simulink model "CurBasedFluxEst_sim"  (R2021b)
settings: Solver=FixedStepAuto  StartTime=0.0  StopTime=SimTime  FixedStep=Ts_sim  MaxStep=Ts_sim  RelTol=1e-3
values from neighbouring files (symbols this model uses):
  FstoWm = 1/PolePairs * 2 * pi    (= 3.14159265359)    [CurBasedFluxEst_param.m]
  Llr = 0.005473    [CurBasedFluxEst_param.m]
  NsToFs = PolePairs/60    (= 0.0333333333333)    [CurBasedFluxEst_param.m]
  PolePairs = 2    [CurBasedFluxEst_param.m]
  RotFluxEst_Ts = Ts_sim    (= 1e-06)    [CurBasedFluxEst_param.m]
  Rr = 0.6258    [CurBasedFluxEst_param.m]
  SVPWM_SampTs = 1/SVPWM_SampFreq    (= 0.001)    [CurBasedFluxEst_param.m]
  SVPWM_SwitchTs = 1/SVPWM_SwitchFreq    (= 5e-05)    [CurBasedFluxEst_param.m]
  Test_NsCntr = 6    [CurBasedFluxEst_param.m]
  Test_NsMax = max(Test_NsArr)    [CurBasedFluxEst_param.m]
  Test_wTs = 1    [CurBasedFluxEst_param.m]
  Tr = Lr / Rr    (= 0.0653131991051)    [CurBasedFluxEst_param.m]
  Ts_sim = 1e-6    (= 1e-06)    [CurBasedFluxEst_param.m]
  Udc = 400    [CurBasedFluxEst_param.m]
  UFCtrl_FWPointFreq = NomFreq    (= 60)    [CurBasedFluxEst_param.m]
  UFCtrl_LinRegPointFreq = 5    [CurBasedFluxEst_param.m]
  UFCtrl_MaxFreq = UFCtrl_FWPointFreq * 2    (= 120)    [CurBasedFluxEst_param.m]
  UFCtrl_Ts = Ts_sim    (= 1e-06)    [CurBasedFluxEst_param.m]
  UFCtrl_UBelowLinReg = 5    [CurBasedFluxEst_param.m]
  UNomLL = 400    [CurBasedFluxEst_param.m]
undefined symbols (not defined in the file or in its folder): NsCntr, Ts_stair
libraries: spsIGBTDiodeLib x6, spsCurrentMeasurementLib x3, spsVoltageMeasurementLib x3, simulink x2, spsAsynchronousMachineSIUnitsLib x1, spsDCVoltageSourceLib x1, spspowerguiLib x1
settings Model: Creator=ArnóczyLászlóVince  LastModifiedBy=ArnóczyLászlóVince

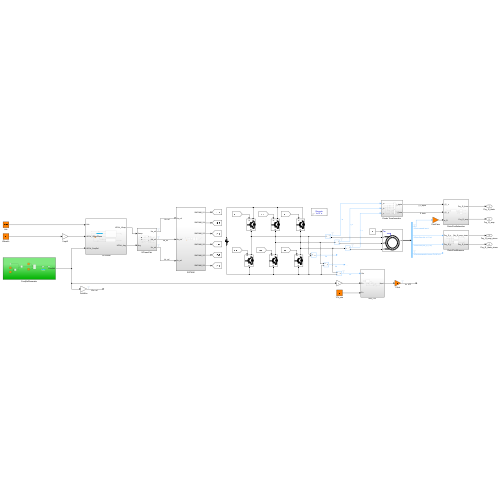
[thumbnail: Simulink's stored preview of the top-level diagram]
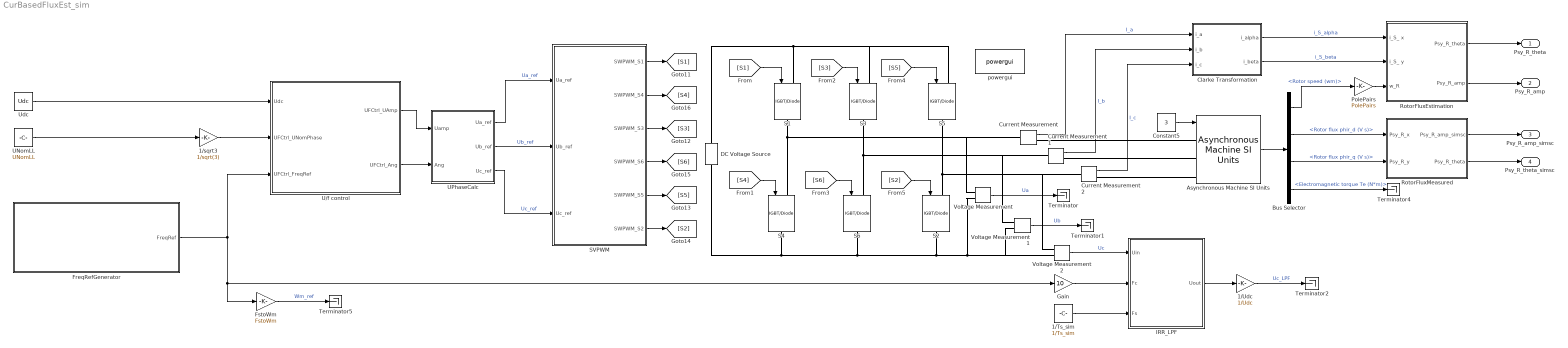
== system CurBasedFluxEst_sim ==
  1/Ts_sim : Constant  Value=1/Ts_sim
  1/Udc : Gain  Gain=1/Udc
  1/sqrt3 : Gain  Gain=1/sqrt(3)
  Asynchronous Machine SI Units : spsAsynchronousMachineSIUnitsLib/Asynchronous Machine SI Units  RotorType=Squirrel-cage  PresetModel=No  MechanicalLoad=Torque Tm  ShowDetailedParameters=on  ReferenceFrame=Stationary  Units=SI  MeasurementBus=off  NominalParameters=[1.845e+04 400 60]  VoltageRatio=1  Stator=[0.5968 0.0003495]  Rotor=[Rr Llr]  Cage1=[0.4155 0.002066]  Cage2=[0.4168 0.0003495]  Lm=Lm  Mechanical=[0.05 0.005879 PolePairs]  PolePairs=PolePairs  InitialConditions=[0 0 0 0 0 0 0 0]  SimulateSaturation=off  Saturation=[14.03593122, 27.81365428, 53.79336849, 72.68890987, 97.98006896, 148.6815601, 215.7428561, 302.9841135, 428.7778367 ; 230, 322, 414, 460, 506, 552, 598, 644, 690]  LoadFlowParameters=1492000  TsPowergui=0  TsBlock=-1  IterativeModel=Trapezoidal non iterative  IterativeDiscreteModel=Trapezoidal non iterative  Pmec=1.492e+006
  Bus Selector : BusSelector  OutputSignals=Mechanical.Rotor speed (wm),Rotor measurements.Rotor flux phir_d (V s),Rotor measurements.Rotor flux phir_q (V s),Mechanical.Electromagnetic torque Te (N*m)
  Clarke Transformation : Subsystem
  Constant5 : Constant  Value=3
  Current Measurement : spsCurrentMeasurementLib/Current Measurement  PhasorSimulation=off  OutputType=Complex  PSBequivalent=0
  Current Measurement1 : spsCurrentMeasurementLib/Current Measurement  PhasorSimulation=off  OutputType=Complex  PSBequivalent=0
  Current Measurement2 : spsCurrentMeasurementLib/Current Measurement  PhasorSimulation=off  OutputType=Complex  PSBequivalent=0
  DC Voltage Source : spsDCVoltageSourceLib/DC Voltage Source  Amplitude=Udc  Measurements=None
  FreqRefGenerator : Subsystem
  FstoWm : Gain  Gain=FstoWm
  Gain : Gain  Gain=10
  IRR_LPF : Subsystem
  PolePairs : Gain  Gain=PolePairs
  RotorFluxEstimation : Subsystem
  RotorFluxMeasured : Subsystem
  S{1..6} (6 alike) : spsIGBTDiodeLib/IGBT//Diode  Ron=1e-3  Rs=1e5  Cs=inf  Measurements=off
  SVPWM : Subsystem
  Terminator{,1..2,4..5} (5 alike) : Terminator
  U/f control : Subsystem
  UNomLL : Constant  Value=UNomLL
  UPhaseCalc : Subsystem
  Udc : Constant  Value=Udc
  Voltage Measurement : spsVoltageMeasurementLib/Voltage Measurement  PhasorSimulation=off  OutputType=Complex  PSBequivalent=0
  Voltage Measurement1 : spsVoltageMeasurementLib/Voltage Measurement  PhasorSimulation=off  OutputType=Complex  PSBequivalent=0
  Voltage Measurement2 : spsVoltageMeasurementLib/Voltage Measurement  PhasorSimulation=off  OutputType=Complex  PSBequivalent=0
  powergui : spspowerguiLib/powergui  Priority=1  SimulationMode=Discrete  SampleTime=Ts_sim  frequency=60  Iterations=50  frequencyindice=0  Pbase=100e6  ErrMax=1e-4  UnitsV=kV  UnitsW=MW  buscounter=0  FunctionMessages=off  echomessages=off  EnableUseOfTLC=off  CurrentSourceSwitches=off  DisableSnubberDevices=off  DisableRonSwitches=off  DisableVfSwitches=off  DisplayEquations=off  AutomaticDiscreteSolvers=off  SolverType=Tustin/Backward Euler (TBE)  Interpol=off  ExternalGateDelay=off  methode=off  Ts=100  x0status=blocks  SPID=on  SwTol=0  HookPort=off  NonlinearTolerance=1e-4  nMaxIteration=100  ContinueOnMaxIteration=off  RestoreLinks=warning  ResistiveCurrentMeasurement=off  Frange=[0:2:500]  Ylog=off  Xlog=on  ShowGrid=off  save=off  variable=ZData  structure=0  ZoomFFT=off  StartTime=0.0  cycles=1  DisplayStyle=1  fundamental=60  FreqAxis=off  MaxFrequency=1000  frequencyindicesteady=1  RmsSteady=1  display=off
  Psy_R_theta : Outport
  Psy_R_amp : Outport  Port=2
  Psy_R_amp_simsc : Outport  Port=3
  Psy_R_theta_simsc : Outport  Port=4
  wires:
  Clarke Transformation/1(i_alpha) -> RotorFluxEstimation/1(i_S_ x)  "i_S_alpha"
  Clarke Transformation/2(i_beta) -> RotorFluxEstimation/2(i_S_ y)  "i_S_beta"
  RotorFluxEstimation/1(Psy_R_theta) -> Psy_R_theta/1
  RotorFluxEstimation/2(Psy_R_amp) -> Psy_R_amp/1
  Asynchronous Machine SI Units/1 -> Bus Selector/1
  Current Measurement/1 -> Clarke Transformation/1(i_a)  "I_a"
  Current Measurement1/1 -> Clarke Transformation/2(i_b)  "I_b"
  Current Measurement2/1 -> Clarke Transformation/3(i_c)  "I_c"
  Bus Selector/1 -> PolePairs/1  "<Rotor speed (wm)>"
  [S1] -> S1/1
  [S4] -> S4/1
  [S3] -> S3/1
  [S6] -> S6/1
  [S5] -> S5/1
  [S2] -> S2/1
  Constant5/1 -> Asynchronous Machine SI Units/1
  Voltage Measurement2/1 -> IRR_LPF/1(Uin)  "Uc"
  Voltage Measurement1/1 -> Terminator1/1  "Ub"
  Voltage Measurement/1 -> Terminator/1  "Ua"
  SVPWM/1(SWPWM_S1) -> [S1]
  SVPWM/2(SWPWM_S4) -> [S4]
  SVPWM/3(SWPWM_S3) -> [S3]
  SVPWM/4(SWPWM_S6) -> [S6]
  SVPWM/5(SWPWM_S5) -> [S5]
  SVPWM/6(SWPWM_S2) -> [S2]
  PolePairs/1 -> RotorFluxEstimation/3(w_R)
  RotorFluxMeasured/1(Psy_R_amp_simsc) -> Psy_R_amp_simsc/1
  RotorFluxMeasured/2(Psy_R_theta) -> Psy_R_theta_simsc/1
  Bus Selector/3 -> RotorFluxMeasured/2(Psy_R_y)  "<Rotor flux phir_q (V s)>"
  Bus Selector/2 -> RotorFluxMeasured/1(Psy_R_x)  "<Rotor flux phir_d (V s)>"
  Bus Selector/4 -> Terminator4/1  "<Electromagnetic torque Te (N*m)>"
  UPhaseCalc/1(Ua_ref) -> SVPWM/1(Ua_ref)  "Ua_ref"
  UPhaseCalc/2(Ub_ref) -> SVPWM/2(Ub_ref)  "Ub_ref"
  UPhaseCalc/3(Uc_ref) -> SVPWM/3(Uc_ref)  "Uc_ref"
  UNomLL/1 -> 1/sqrt3/1
  FstoWm/1 -> Terminator5/1  "Wm_ref"
  U/f control/1(UFCtrl_UAmp) -> UPhaseCalc/1(Uamp)
  U/f control/2(UFCtrl_Ang) -> UPhaseCalc/2(Ang)
  1/sqrt3/1 -> U/f control/2(UFCtrl_UNomPhase)
  Udc/1 -> U/f control/1(Udc)
  FreqRefGenerator/1(FreqRef) -> U/f control/3(UFCtrl_FreqRef), FstoWm/1, Gain/1
  Gain/1 -> IRR_LPF/2(Fc)
  IRR_LPF/1(Uout) -> 1/Udc/1
  1/Udc/1 -> Terminator2/1  "Uc_LPF"
  1/Ts_sim/1 -> IRR_LPF/3(Fs)
  connections:
  Asynchronous Machine SI Units/LConn1 -- Current Measurement/RConn1
  S3/RConn1 -- Current Measurement1/LConn1 -- Voltage Measurement1/LConn1 -- S6/LConn1
  S4/LConn1 -- Current Measurement/LConn1 -- Voltage Measurement/LConn1 -- S1/RConn1
  S2/LConn1 -- Current Measurement2/LConn1 -- Voltage Measurement2/LConn1 -- S5/RConn1
  DC Voltage Source/RConn1 -- S1/LConn1 -- S3/LConn1 -- S5/LConn1
  DC Voltage Source/LConn1 -- Voltage Measurement2/LConn2 -- Voltage Measurement1/LConn2 -- Voltage Measurement/LConn2 -- S2/RConn1 -- S6/RConn1 -- S4/RConn1
  Asynchronous Machine SI Units/LConn3 -- Current Measurement2/RConn1
  Asynchronous Machine SI Units/LConn2 -- Current Measurement1/RConn1

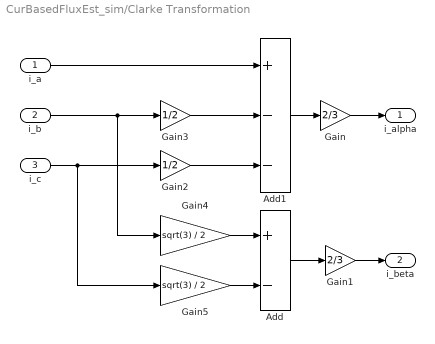
== system CurBasedFluxEst_sim/Clarke Transformation ==
  i_a : Inport
  i_b : Inport  Port=2
  i_c : Inport  Port=3
  Add : Sum  Inputs=+-
  Add1 : Sum  Inputs=+--
  Gain : Gain  Gain=2/3
  Gain1 : Gain  Gain=2/3
  Gain2 : Gain  Gain=1/2
  Gain3 : Gain  Gain=1/2
  Gain4 : Gain  Gain=sqrt(3) / 2
  Gain5 : Gain  Gain=sqrt(3) / 2
  i_alpha : Outport
  i_beta : Outport  Port=2
  wires:
  Gain4/1 -> Add/1
  Add/1 -> Gain1/1
  i_a/1 -> Add1/1
  Gain5/1 -> Add/2
  Add1/1 -> Gain/1
  Gain2/1 -> Add1/3
  Gain3/1 -> Add1/2
  i_b/1 -> Gain4/1, Gain3/1
  i_c/1 -> Gain5/1, Gain2/1
  Gain1/1 -> i_beta/1
  Gain/1 -> i_alpha/1

== system CurBasedFluxEst_sim/FreqRefGenerator ==
  note: Nr = ~ Ns
  Clock : Clock
  NrToFs : Gain  Gain=NsToFs
  Product : Product
  Relational Operator : RelationalOperator  OutDataTypeStr=boolean  RndMeth=Simplest
  Switch : Switch  Criteria=u2 ~= 0  Threshold=Ts_stair * NsCntr
  Test_NsArr : simulink/Sources/Repeating Sequence Stair  OutValues=Test_NsArr  tsamp=Test_wTs  OutMin=[]  OutMax=[]  OutDataTypeStr=double  OutputDataTypeScalingMode=double  OutDataType=fixdt(0,8)  ConRadixGroup=Best Precision: Vector-wise  OutScaling=2^-12
  Test_NsCntr : Constant  Value=Test_NsCntr
  Test_NsMax : Constant  Value=Test_NsMax
  Test_wTs : Constant  Value=Test_wTs
  FreqRef : Outport
  wires:
  Clock/1 -> Relational Operator/1
  Test_NsArr/1 -> Switch/3
  Test_NsCntr/1 -> Product/2
  Switch/1 -> NrToFs/1  "Nr_ref"
  Product/1 -> Relational Operator/2
  Test_NsMax/1 -> Switch/1
  Test_wTs/1 -> Product/1
  Relational Operator/1 -> Switch/2
  NrToFs/1 -> FreqRef/1

== system CurBasedFluxEst_sim/IRR_LPF ==
  Uin : Inport
  Fc : Inport  Port=2
  Fs : Inport  Port=3
  Add6 : Sum  Inputs=+-
  Add7 : Sum
  MATLAB Function : MATLAB Function  TreatAsAtomicUnit=on
  Product3 : Product
  Unit Delay3 : UnitDelay  SampleTime=-1  HasFrameUpgradeWarning=on
  Uout : Outport
  wires:
  Add6/1 -> Product3/2
  Product3/1 -> Add7/1
  MATLAB Function/1(alpha) -> Product3/1
  Unit Delay3/1 -> Add7/2, Add6/2
  Add7/1 -> Uout/1, Unit Delay3/1
  Uin/1 -> Add6/1
  Fc/1 -> MATLAB Function/1(Fc)
  Fs/1 -> MATLAB Function/2(Fs)

== system CurBasedFluxEst_sim/RotorFluxEstimation ==
  i_S_ x : Inport
  i_S_ y : Inport  Port=2
  w_R : Inport  Port=3
  PsyR_Amp_Calc : Subsystem
  PsyR_Amp_angle : Subsystem
  PsyR_XY_calc : Subsystem
  Psy_R_theta : Outport
  Psy_R_amp : Outport  Port=2
  wires:
  w_R/1 -> PsyR_XY_calc/2(w_R)
  i_S_ y/1 -> PsyR_XY_calc/3(i_S_ y)
  i_S_ x/1 -> PsyR_XY_calc/1(i_S_ x)
  PsyR_Amp_Calc/1(Psy_R_amp) -> Psy_R_amp/1
  PsyR_Amp_angle/1(Psy_R_theta) -> Psy_R_theta/1
  PsyR_XY_calc/1(Psy_R_ x) -> PsyR_Amp_Calc/1(Psy_R_ x), PsyR_Amp_angle/1(Psy_R_ x)
  PsyR_XY_calc/2(Psy_R_ y) -> PsyR_Amp_Calc/2(Psy_R_ y), PsyR_Amp_angle/2(Psy_R_ y)

== system CurBasedFluxEst_sim/RotorFluxMeasured ==
  Psy_R_x : Inport
  Psy_R_y : Inport  Port=2
  PsyR_Amp_Calc : Subsystem
  PsyR_Amp_angle : Subsystem
  Psy_R_amp_simsc : Outport
  Psy_R_theta : Outport  Port=2
  wires:
  PsyR_Amp_angle/1(Psy_R_theta) -> Psy_R_theta/1
  PsyR_Amp_Calc/1(Psy_R_amp_simsc) -> Psy_R_amp_simsc/1
  Psy_R_x/1 -> PsyR_Amp_Calc/1(Psy_x), PsyR_Amp_angle/1(Psy_R_ x)
  Psy_R_y/1 -> PsyR_Amp_Calc/2(Psy_y), PsyR_Amp_angle/2(Psy_R_ y)

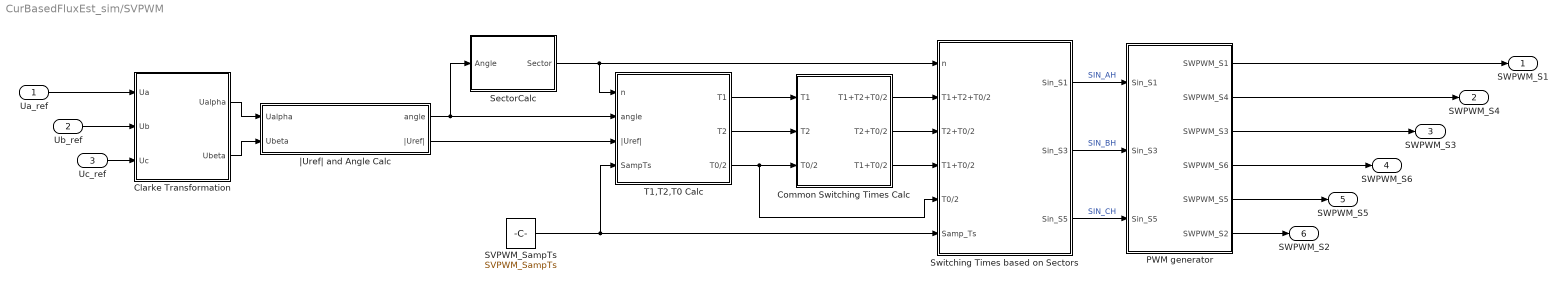
== system CurBasedFluxEst_sim/SVPWM ==
  Ua_ref : Inport
  Ub_ref : Inport  Port=2
  Uc_ref : Inport  Port=3
  " SectorCalc" : Subsystem
  Clarke Transformation : Subsystem
  Common Switching Times Calc : Subsystem
  PWM generator : Subsystem
  SVPWM_SampTs : Constant  Value=SVPWM_SampTs
  "Switching Times based on Sectors " : Subsystem
  T1,T2,T0 Calc : Subsystem
  |Uref| and Angle Calc : Subsystem
  SWPWM_S1 : Outport
  SWPWM_S4 : Outport  Port=2
  SWPWM_S3 : Outport  Port=3
  SWPWM_S6 : Outport  Port=4
  SWPWM_S5 : Outport  Port=5
  SWPWM_S2 : Outport  Port=6
  wires:
  " SectorCalc"/1(Sector) -> T1,T2,T0 Calc/1(n), "Switching Times based on Sectors "/1(n)
  SVPWM_SampTs/1 -> T1,T2,T0 Calc/4(SampTs), "Switching Times based on Sectors "/6(Samp_Ts)
  "Switching Times based on Sectors "/3(Sin_S5) -> PWM generator/3(Sin_S5)  "SIN_CH"
  PWM generator/2(SWPWM_S4) -> SWPWM_S4/1
  T1,T2,T0 Calc/1(T1) -> Common Switching Times Calc/1(T1)
  "Switching Times based on Sectors "/2(Sin_S3) -> PWM generator/2(Sin_S3)  "SIN_BH"
  Common Switching Times Calc/2(T2+T0/2) -> "Switching Times based on Sectors "/3(T2+T0/2)
  Common Switching Times Calc/3(T1+T0/2) -> "Switching Times based on Sectors "/4(T1+T0/2)
  |Uref| and Angle Calc/1(angle) -> T1,T2,T0 Calc/2(angle), " SectorCalc"/1(Angle)
  |Uref| and Angle Calc/2(|Uref|) -> T1,T2,T0 Calc/3(|Uref|)
  "Switching Times based on Sectors "/1(Sin_S1) -> PWM generator/1(Sin_S1)  "SIN_AH"
  T1,T2,T0 Calc/2(T2) -> Common Switching Times Calc/2(T2)
  Common Switching Times Calc/1(T1+T2+T0/2) -> "Switching Times based on Sectors "/2(T1+T2+T0/2)
  PWM generator/3(SWPWM_S3) -> SWPWM_S3/1
  PWM generator/4(SWPWM_S6) -> SWPWM_S6/1
  Ua_ref/1 -> Clarke Transformation/1(Ua)
  PWM generator/6(SWPWM_S2) -> SWPWM_S2/1
  PWM generator/5(SWPWM_S5) -> SWPWM_S5/1
  PWM generator/1(SWPWM_S1) -> SWPWM_S1/1
  Ub_ref/1 -> Clarke Transformation/2(Ub)
  T1,T2,T0 Calc/3(T0/2) -> "Switching Times based on Sectors "/5(T0/2), Common Switching Times Calc/3(T0/2)
  Clarke Transformation/2(Ubeta) -> |Uref| and Angle Calc/2(Ubeta)
  Uc_ref/1 -> Clarke Transformation/3(Uc)
  Clarke Transformation/1(Ualpha) -> |Uref| and Angle Calc/1(Ualpha)

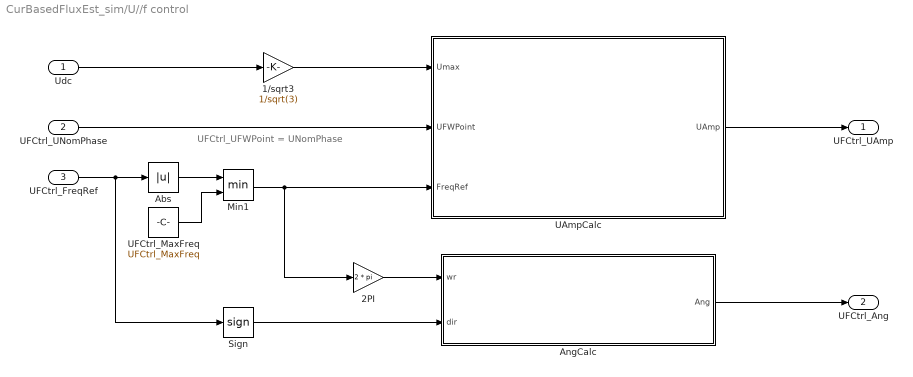
== system CurBasedFluxEst_sim/U//f control ==
  note: UFCtrl_UFWPoint = UNomPhase
  Udc : Inport
  UFCtrl_UNomPhase : Inport  Port=2
  UFCtrl_FreqRef : Inport  Port=3
  1/sqrt3 : Gain  Gain=1/sqrt(3)
  2PI : Gain  Gain=2 * pi
  Abs : Abs
  AngCalc : Subsystem
  Min1 : MinMax  Inputs=2
  Sign : Signum
  UAmpCalc : Subsystem
  UFCtrl_MaxFreq : Constant  Value=UFCtrl_MaxFreq
  UFCtrl_UAmp : Outport
  UFCtrl_Ang : Outport  Port=2
  wires:
  UFCtrl_UNomPhase/1 -> UAmpCalc/2(UFWPoint)
  UAmpCalc/1(UAmp) -> UFCtrl_UAmp/1
  AngCalc/1(Ang) -> UFCtrl_Ang/1
  2PI/1 -> AngCalc/1(wr)
  UFCtrl_MaxFreq/1 -> Min1/2
  Abs/1 -> Min1/1
  Min1/1 -> 2PI/1, UAmpCalc/3(FreqRef)
  UFCtrl_FreqRef/1 -> Sign/1, Abs/1
  Sign/1 -> AngCalc/2(dir)
  Udc/1 -> 1/sqrt3/1
  1/sqrt3/1 -> UAmpCalc/1(Umax)

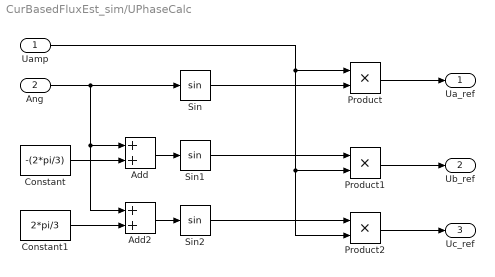
== system CurBasedFluxEst_sim/UPhaseCalc ==
  Uamp : Inport
  Ang : Inport  Port=2
  Add : Sum
  Add2 : Sum
  Constant : Constant  Value=-(2*pi/3)
  Constant1 : Constant  Value=2*pi/3
  Product : Product
  Product1 : Product
  Product2 : Product
  Sin : Trigonometry
  Sin1 : Trigonometry
  Sin2 : Trigonometry
  Ua_ref : Outport
  Ub_ref : Outport  Port=2
  Uc_ref : Outport  Port=3
  wires:
  Product/1 -> Ua_ref/1
  Uamp/1 -> Product2/2, Product1/2, Product/1
  Product2/1 -> Uc_ref/1
  Ang/1 -> Sin/1, Add/1, Add2/1
  Constant/1 -> Add/2
  Constant1/1 -> Add2/2
  Sin/1 -> Product/2
  Add2/1 -> Sin2/1
  Add/1 -> Sin1/1
  Sin1/1 -> Product1/1
  Sin2/1 -> Product2/1
  Product1/1 -> Ub_ref/1

== system CurBasedFluxEst_sim/RotorFluxEstimation/PsyR_Amp_Calc ==
  Psy_R_ x : Inport
  Psy_R_ y : Inport  Port=2
  Add2 : Sum
  Sqrt : Sqrt  SaturateOnIntegerOverflow=on
  Square : Math  Operator=square  SaturateOnIntegerOverflow=on
  Square1 : Math  Operator=square  SaturateOnIntegerOverflow=on
  Psy_R_amp : Outport
  wires:
  Psy_R_ y/1 -> Square/1
  Square/1 -> Add2/1
  Psy_R_ x/1 -> Square1/1
  Square1/1 -> Add2/2
  Add2/1 -> Sqrt/1
  Sqrt/1 -> Psy_R_amp/1

== system CurBasedFluxEst_sim/RotorFluxEstimation/PsyR_Amp_angle ==
  Psy_R_ x : Inport
  Psy_R_ y : Inport  Port=2
  Tan : Trigonometry  Operator=atan2
  Psy_R_theta : Outport
  wires:
  Psy_R_ y/1 -> Tan/1
  Tan/1 -> Psy_R_theta/1
  Psy_R_ x/1 -> Tan/2

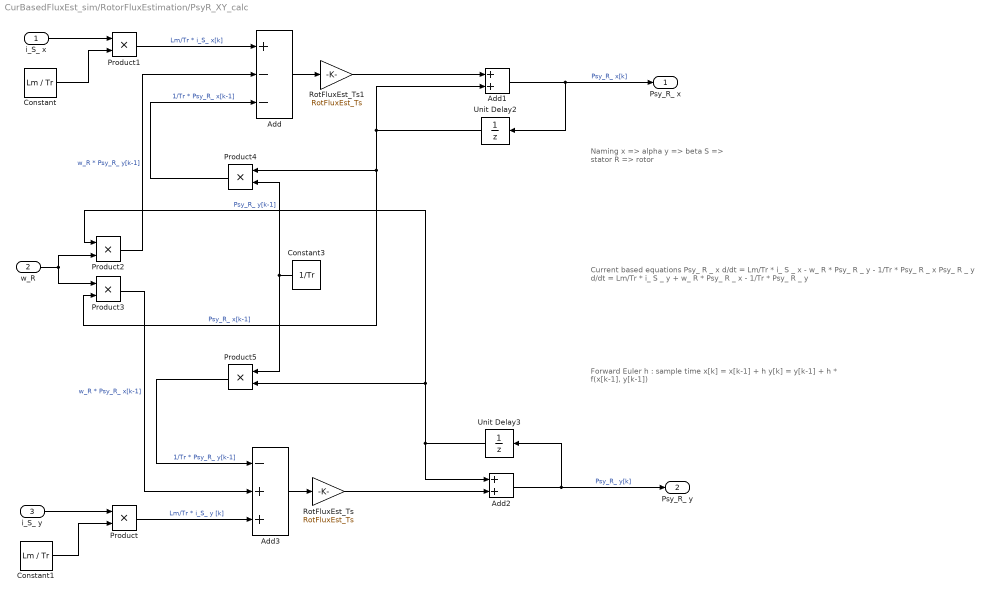
== system CurBasedFluxEst_sim/RotorFluxEstimation/PsyR_XY_calc ==
  note: Forward Euler
      | h : sample time
      | x[k] = x[k-1] + h
      | y[k] = y[k-1] + h * f(x[k-1], y[k-1])
  note: Current based equations
      | Psy_ R _ x d/dt = Lm/Tr * i_ S _ x - w_ R * Psy_ R _ y - 1/Tr * Psy_ R _ x
      | Psy_ R _ y d/dt = Lm/Tr * i_ S _ y + w_ R * Psy_ R _ x - 1/Tr * Psy_ R _ y
  note: Naming
      |
      | x => alpha
      | y => beta
      | S => stator
      | R => rotor
  i_S_ x : Inport
  w_R : Inport  Port=2
  i_S_ y : Inport  Port=3
  Add : Sum  Inputs=+--
  Add1 : Sum
  Add2 : Sum
  Add3 : Sum  Inputs=-++
  Constant : Constant  Value=Lm / Tr
  Constant1 : Constant  Value=Lm / Tr
  Constant3 : Constant  Value=1/Tr
  Product{,1..5} (6 alike) : Product
  RotFluxEst_Ts : Gain  Gain=RotFluxEst_Ts
  RotFluxEst_Ts1 : Gain  Gain=RotFluxEst_Ts
  Unit Delay2 : UnitDelay  SampleTime=-1  HasFrameUpgradeWarning=on
  Unit Delay3 : UnitDelay  SampleTime=-1  HasFrameUpgradeWarning=on
  Psy_R_ x : Outport
  Psy_R_ y : Outport  Port=2
  wires:
  Unit Delay2/1 -> Product4/1, Product3/2, Add1/2  "Psy_R_ x[k-1]"
  Add3/1 -> RotFluxEst_Ts/1
  w_R/1 -> Product3/1, Product2/2
  Constant1/1 -> Product/2
  i_S_ y/1 -> Product/1
  Product2/1 -> Add/2  "w_R * Psy_R_ y[k-1]"
  Add/1 -> RotFluxEst_Ts1/1
  Product1/1 -> Add/1  "Lm/Tr * i_S_ x[k]"
  Product4/1 -> Add/3  "1/Tr * Psy_R_ x[k-1]"
  Constant3/1 -> Product5/1, Product4/2
  Product5/1 -> Add3/1  "1/Tr * Psy_R_ y[k-1]"
  Product3/1 -> Add3/2  "w_R * Psy_R_ x[k-1]"
  Product/1 -> Add3/3  "Lm/Tr * i_S_ y [k]"
  i_S_ x/1 -> Product1/1
  Constant/1 -> Product1/2
  Add1/1 -> Psy_R_ x/1, Unit Delay2/1  "Psy_R_ x[k]"
  Add2/1 -> Psy_R_ y/1, Unit Delay3/1  "Psy_R_ y[k]"
  Unit Delay3/1 -> Product5/2, Product2/1, Add2/1  "Psy_R_ y[k-1]"
  RotFluxEst_Ts/1 -> Add2/2
  RotFluxEst_Ts1/1 -> Add1/1

== system CurBasedFluxEst_sim/RotorFluxMeasured/PsyR_Amp_Calc ==
  Psy_x : Inport
  Psy_y : Inport  Port=2
  Add2 : Sum
  Sqrt : Sqrt  SaturateOnIntegerOverflow=on
  Square : Math  Operator=square  SaturateOnIntegerOverflow=on
  Square1 : Math  Operator=square  SaturateOnIntegerOverflow=on
  Psy_R_amp_simsc : Outport
  wires:
  Add2/1 -> Sqrt/1
  Square/1 -> Add2/1
  Square1/1 -> Add2/2
  Psy_y/1 -> Square1/1
  Sqrt/1 -> Psy_R_amp_simsc/1
  Psy_x/1 -> Square/1

== system CurBasedFluxEst_sim/RotorFluxMeasured/PsyR_Amp_angle ==
  Psy_R_ x : Inport
  Psy_R_ y : Inport  Port=2
  Tan : Trigonometry  Operator=atan2
  Psy_R_theta : Outport
  wires:
  Psy_R_ y/1 -> Tan/1
  Tan/1 -> Psy_R_theta/1
  Psy_R_ x/1 -> Tan/2

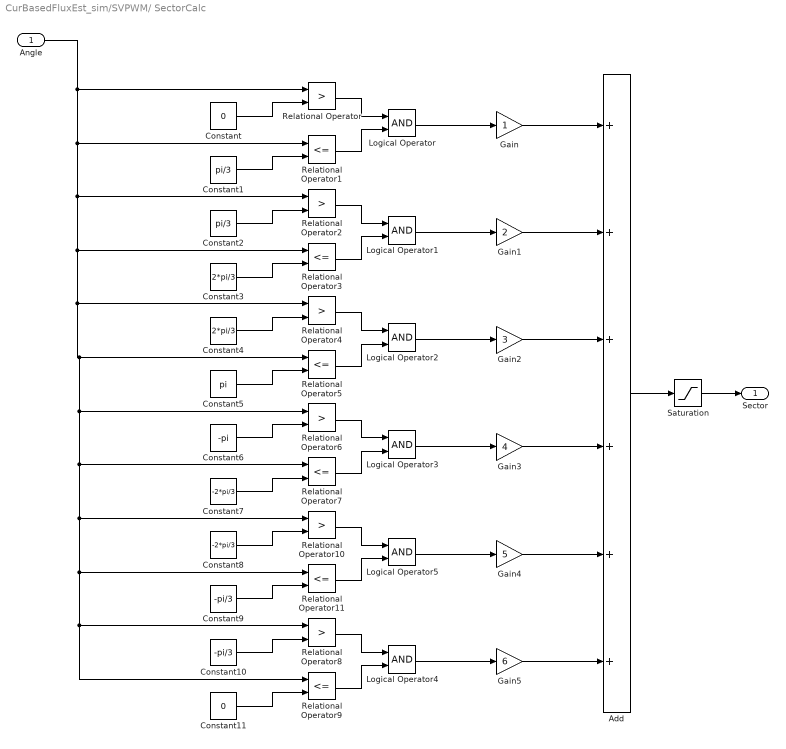
== system CurBasedFluxEst_sim/SVPWM/ SectorCalc ==
  Angle : Inport
  Add : Sum  Inputs=++++++
  Constant : Constant  Value=0
  Constant1 : Constant  Value=pi/3
  Constant10 : Constant  Value=-pi/3
  Constant11 : Constant  Value=0
  Constant2 : Constant  Value=pi/3
  Constant3 : Constant  Value=2*pi/3
  Constant4 : Constant  Value=2*pi/3
  Constant5 : Constant  Value=pi
  Constant6 : Constant  Value=-pi
  Constant7 : Constant  Value=-2*pi/3
  Constant8 : Constant  Value=-2*pi/3
  Constant9 : Constant  Value=-pi/3
  Gain : Gain
  Gain1 : Gain  Gain=2
  Gain2 : Gain  Gain=3
  Gain3 : Gain  Gain=4
  Gain4 : Gain  Gain=5
  Gain5 : Gain  Gain=6
  Logical Operator{,1..5} (6 alike) : Logic  AllPortsSameDT=off  OutDataTypeStr=boolean
  Relational Operator{,2,4,6,8,10} (6 alike) : RelationalOperator  Operator=>  OutDataTypeStr=boolean  RndMeth=Simplest
  Relational Operator{1,3,5,7,9,11} (6 alike) : RelationalOperator  Operator=<=  OutDataTypeStr=boolean  RndMeth=Simplest
  Saturation : Saturate  UpperLimit=6  LowerLimit=1
  Sector : Outport
  wires:
  Relational Operator/1 -> Logical Operator/1
  Relational Operator1/1 -> Logical Operator/2
  Angle/1 -> Relational Operator9/1, Relational Operator8/1, Relational Operator11/1, Relational Operator10/1, Relational Operator7/1, Relational Operator6/1, Relational Operator5/1, Relational Operator4/1, Relational Operator3/1, Relational Operator2/1, Relational Operator1/1, Relational Operator/1
  Relational Operator2/1 -> Logical Operator1/1
  Relational Operator3/1 -> Logical Operator1/2
  Relational Operator4/1 -> Logical Operator2/1
  Relational Operator5/1 -> Logical Operator2/2
  Relational Operator6/1 -> Logical Operator3/1
  Relational Operator7/1 -> Logical Operator3/2
  Relational Operator8/1 -> Logical Operator4/1
  Relational Operator9/1 -> Logical Operator4/2
  Relational Operator10/1 -> Logical Operator5/1
  Relational Operator11/1 -> Logical Operator5/2
  Logical Operator/1 -> Gain/1
  Logical Operator1/1 -> Gain1/1
  Logical Operator2/1 -> Gain2/1
  Logical Operator3/1 -> Gain3/1
  Logical Operator5/1 -> Gain4/1
  Logical Operator4/1 -> Gain5/1
  Gain/1 -> Add/1
  Gain1/1 -> Add/2
  Gain2/1 -> Add/3
  Gain3/1 -> Add/4
  Gain4/1 -> Add/5
  Gain5/1 -> Add/6
  Constant/1 -> Relational Operator/2
  Constant1/1 -> Relational Operator1/2
  Constant2/1 -> Relational Operator2/2
  Constant3/1 -> Relational Operator3/2
  Constant4/1 -> Relational Operator4/2
  Constant5/1 -> Relational Operator5/2
  Constant6/1 -> Relational Operator6/2
  Constant7/1 -> Relational Operator7/2
  Constant8/1 -> Relational Operator10/2
  Constant9/1 -> Relational Operator11/2
  Constant10/1 -> Relational Operator8/2
  Constant11/1 -> Relational Operator9/2
  Add/1 -> Saturation/1
  Saturation/1 -> Sector/1

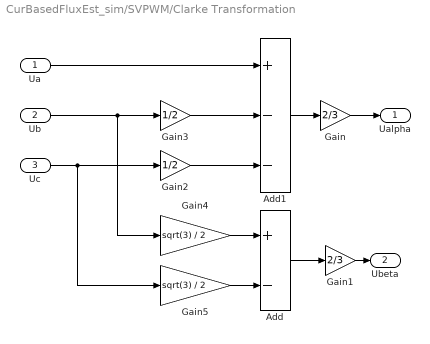
== system CurBasedFluxEst_sim/SVPWM/Clarke Transformation ==
  Ua : Inport
  Ub : Inport  Port=2
  Uc : Inport  Port=3
  Add : Sum  Inputs=+-
  Add1 : Sum  Inputs=+--
  Gain : Gain  Gain=2/3
  Gain1 : Gain  Gain=2/3
  Gain2 : Gain  Gain=1/2
  Gain3 : Gain  Gain=1/2
  Gain4 : Gain  Gain=sqrt(3) / 2
  Gain5 : Gain  Gain=sqrt(3) / 2
  Ualpha : Outport
  Ubeta : Outport  Port=2
  wires:
  Gain3/1 -> Add1/2
  Gain5/1 -> Add/2
  Gain4/1 -> Add/1
  Gain2/1 -> Add1/3
  Gain/1 -> Ualpha/1
  Uc/1 -> Gain5/1, Gain2/1
  Ub/1 -> Gain4/1, Gain3/1
  Ua/1 -> Add1/1
  Add/1 -> Gain1/1
  Add1/1 -> Gain/1
  Gain1/1 -> Ubeta/1

== system CurBasedFluxEst_sim/SVPWM/Common Switching Times Calc ==
  T1 : Inport
  T2 : Inport  Port=2
  T0/2 : Inport  Port=3
  Add : Sum
  Add1 : Sum
  Add3 : Sum
  T1+T2+T0/2 : Outport
  T2+T0/2 : Outport  Port=2
  T1+T0/2 : Outport  Port=3
  wires:
  Add/1 -> T2+T0/2/1, Add3/2
  Add1/1 -> T1+T0/2/1
  Add3/1 -> T1+T2+T0/2/1
  T1/1 -> Add3/1, Add1/1
  T2/1 -> Add/2
  T0/2/1 -> Add/1, Add1/2

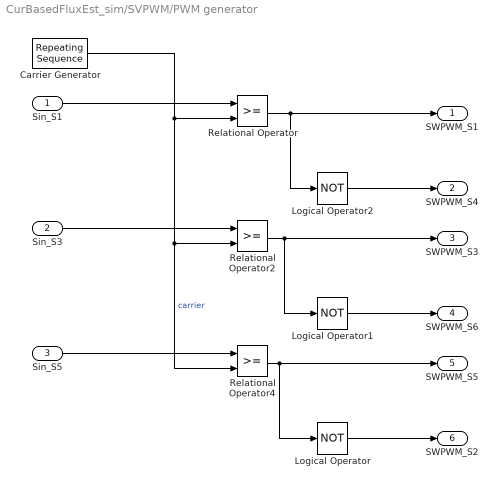
== system CurBasedFluxEst_sim/SVPWM/PWM generator ==
  Sin_S1 : Inport
  Sin_S3 : Inport  Port=2
  Sin_S5 : Inport  Port=3
  Carrier Generator : simulink/Sources/Repeating Sequence  rep_seq_t="[0  SVPWM_SwitchTs/2 SVPWM_SwitchTs ]"  rep_seq_y="[  0 1 0 ]"
  Logical Operator : Logic  Operator=NOT  AllPortsSameDT=off  OutDataTypeStr=boolean
  Logical Operator1 : Logic  Operator=NOT  AllPortsSameDT=off  OutDataTypeStr=boolean
  Logical Operator2 : Logic  Operator=NOT  AllPortsSameDT=off  OutDataTypeStr=boolean
  Relational Operator : RelationalOperator  OutDataTypeStr=boolean  RndMeth=Simplest
  Relational Operator2 : RelationalOperator  OutDataTypeStr=boolean  RndMeth=Simplest
  Relational Operator4 : RelationalOperator  OutDataTypeStr=boolean  RndMeth=Simplest
  SWPWM_S1 : Outport
  SWPWM_S4 : Outport  Port=2
  SWPWM_S3 : Outport  Port=3
  SWPWM_S6 : Outport  Port=4
  SWPWM_S5 : Outport  Port=5
  SWPWM_S2 : Outport  Port=6
  wires:
  Sin_S1/1 -> Relational Operator/1
  Sin_S3/1 -> Relational Operator2/1
  Sin_S5/1 -> Relational Operator4/1
  Relational Operator/1 -> Logical Operator2/1, SWPWM_S1/1
  Relational Operator2/1 -> SWPWM_S3/1, Logical Operator1/1
  Relational Operator4/1 -> SWPWM_S5/1, Logical Operator/1
  Logical Operator1/1 -> SWPWM_S6/1
  Logical Operator2/1 -> SWPWM_S4/1
  Logical Operator/1 -> SWPWM_S2/1
  Carrier Generator/1 -> Relational Operator4/2, Relational Operator2/2, Relational Operator/2  "carrier"

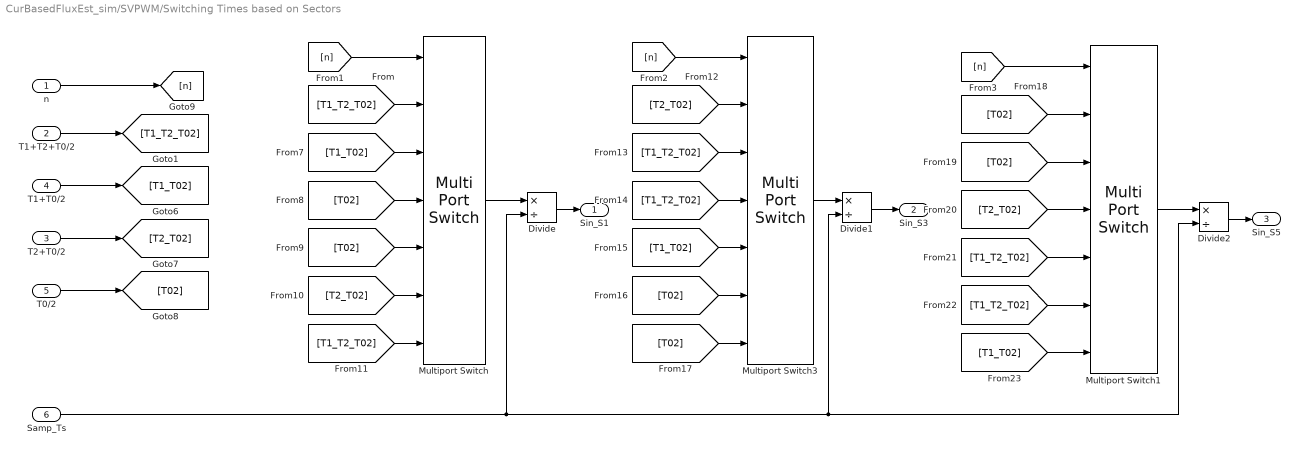
== system CurBasedFluxEst_sim/SVPWM/Switching Times based on Sectors  ==
  n : Inport
  T1+T2+T0/2 : Inport  Port=2
  T2+T0/2 : Inport  Port=3
  T1+T0/2 : Inport  Port=4
  T0/2 : Inport  Port=5
  Samp_Ts : Inport  Port=6
  Divide : Product  Inputs=*/
  Divide1 : Product  Inputs=*/
  Divide2 : Product  Inputs=*/
  Multiport Switch : MultiPortSwitch  DataPortOrder=Specify indices  Inputs=6  DataPortIndices={1,2,3,4,5,6}  DiagnosticForDefault=None
  Multiport Switch1 : MultiPortSwitch  DataPortOrder=Specify indices  Inputs=6  DataPortIndices={1,2,3,4,5,6}  DiagnosticForDefault=None
  Multiport Switch3 : MultiPortSwitch  DataPortOrder=Specify indices  Inputs=6  DataPortIndices={1,2,3,4,5,6}  DiagnosticForDefault=None
  Sin_S1 : Outport
  Sin_S3 : Outport  Port=2
  Sin_S5 : Outport  Port=3
  wires:
  [n] -> Multiport Switch/1
  [n] -> Multiport Switch3/1
  [T1_T2_T02] -> Multiport Switch/7
  [T1_T2_T02] -> Multiport Switch3/3
  [T02] -> Multiport Switch/4
  [T02] -> Multiport Switch/5
  [T1_T2_T02] -> Multiport Switch/2
  [T1_T2_T02] -> Multiport Switch3/4
  [T02] -> Multiport Switch3/7
  [T1_T02] -> Multiport Switch1/7
  [T2_T02] -> Multiport Switch1/4
  [T02] -> Multiport Switch1/3
  [T1_T02] -> Multiport Switch3/5
  [T1_T2_T02] -> Multiport Switch1/5
  [T2_T02] -> Multiport Switch3/2
  [T02] -> Multiport Switch1/2
  [T1_T02] -> Multiport Switch/3
  [T2_T02] -> Multiport Switch/6
  [T02] -> Multiport Switch3/6
  [T1_T2_T02] -> Multiport Switch1/6
  [n] -> Multiport Switch1/1
  n/1 -> [n]
  T1+T2+T0/2/1 -> [T1_T2_T02]
  T1+T0/2/1 -> [T1_T02]
  T2+T0/2/1 -> [T2_T02]
  T0/2/1 -> [T02]
  Samp_Ts/1 -> Divide/2, Divide2/2, Divide1/2
  Divide/1 -> Sin_S1/1
  Multiport Switch/1 -> Divide/1
  Multiport Switch3/1 -> Divide1/1
  Divide1/1 -> Sin_S3/1
  Divide2/1 -> Sin_S5/1
  Multiport Switch1/1 -> Divide2/1

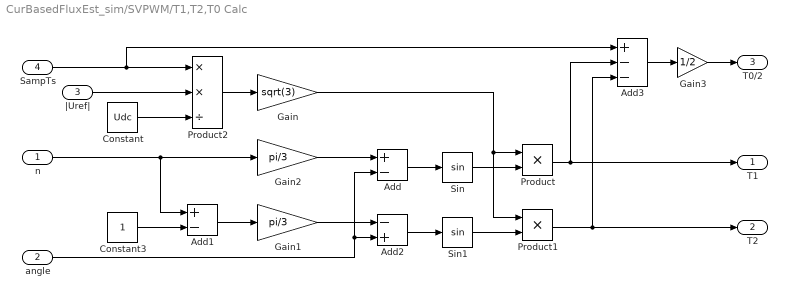
== system CurBasedFluxEst_sim/SVPWM/T1,T2,T0 Calc ==
  n : Inport
  angle : Inport  Port=2
  |Uref| : Inport  Port=3
  SampTs : Inport  Port=4
  Add : Sum  Inputs=+-
  Add1 : Sum  Inputs=+-
  Add2 : Sum  Inputs=-+
  Add3 : Sum  Inputs=+--
  Constant : Constant  Value=Udc
  Constant3 : Constant
  Gain : Gain  Gain=sqrt(3)
  Gain1 : Gain  Gain=pi/3
  Gain2 : Gain  Gain=pi/3
  Gain3 : Gain  Gain=1/2
  Product : Product
  Product1 : Product
  Product2 : Product  Inputs=**/
  Sin : Trigonometry
  Sin1 : Trigonometry
  T1 : Outport
  T2 : Outport  Port=2
  T0/2 : Outport  Port=3
  wires:
  |Uref|/1 -> Product2/2
  Gain2/1 -> Add/1
  Add/1 -> Sin/1
  Product2/1 -> Gain/1
  Sin/1 -> Product/2
  Product/1 -> T1/1, Add3/2
  Sin1/1 -> Product1/2
  n/1 -> Gain2/1, Add1/1
  Add1/1 -> Gain1/1
  Constant3/1 -> Add1/2
  Add2/1 -> Sin1/1
  Product1/1 -> T2/1, Add3/3
  Add3/1 -> Gain3/1
  SampTs/1 -> Add3/1, Product2/1
  Gain/1 -> Product/1, Product1/1
  angle/1 -> Add/2, Add2/2
  Gain1/1 -> Add2/1
  Gain3/1 -> T0/2/1
  Constant/1 -> Product2/3

== system CurBasedFluxEst_sim/SVPWM/|Uref| and Angle Calc ==
  Ualpha : Inport
  Ubeta : Inport  Port=2
  Add : Sum
  Sqrt : Sqrt  SaturateOnIntegerOverflow=on
  Square : Math  Operator=square  OutputSignalType=real  SaturateOnIntegerOverflow=on
  Square1 : Math  Operator=square  OutputSignalType=real  SaturateOnIntegerOverflow=on
  Trigonometric Function : Trigonometry  Operator=atan2
  angle : Outport
  |Uref| : Outport  Port=2
  wires:
  Sqrt/1 -> |Uref|/1  "vref"
  Trigonometric Function/1 -> angle/1  "angle"
  Ualpha/1 -> Square/1, Trigonometric Function/2
  Ubeta/1 -> Trigonometric Function/1, Square1/1
  Square/1 -> Add/1
  Square1/1 -> Add/2
  Add/1 -> Sqrt/1

== system CurBasedFluxEst_sim/U//f control/AngCalc ==
  wr : Inport
  dir : Inport  Port=2
  Add : Sum
  Product : Product
  UFCtrl_Ts : Gain  Gain=UFCtrl_Ts
  Unit Delay : UnitDelay  SampleTime=-1  HasFrameUpgradeWarning=on
  angWrapper : Subsystem
  Ang : Outport
  wires:
  Unit Delay/1 -> Add/2
  UFCtrl_Ts/1 -> Add/1
  wr/1 -> UFCtrl_Ts/1
  Add/1 -> angWrapper/1(angIn)  "wt"
  angWrapper/1(angOut) -> Unit Delay/1, Product/2
  dir/1 -> Product/1
  Product/1 -> Ang/1

== system CurBasedFluxEst_sim/U//f control/UAmpCalc ==
  Umax : Inport
  UFWPoint : Inport  Port=2
  FreqRef : Inport  Port=3
  BelowFWPoint : Subsystem
  Constant : Constant  Value=0
  Constant1 : Constant  Value=-1
  Constant2 : Constant
  Min : MinMax  Inputs=2
  Product : Product
  Relational Operator : RelationalOperator  Operator=>  OutDataTypeStr=boolean  RndMeth=Simplest
  Switch : Switch  Criteria=u2 ~= 0  Threshold=Ts_stair * NsCntr
  UAmp : Outport
  wires:
  Constant1/1 -> Switch/3
  Constant2/1 -> Switch/1
  Relational Operator/1 -> Switch/2
  BelowFWPoint/1(Uamp) -> Min/2
  Switch/1 -> Product/1
  Constant/1 -> Relational Operator/2
  UFWPoint/1 -> BelowFWPoint/2(UFWPoint)
  Umax/1 -> Min/1
  Min/1 -> Product/2
  Product/1 -> UAmp/1
  FreqRef/1 -> BelowFWPoint/1(FreqRef), Relational Operator/1

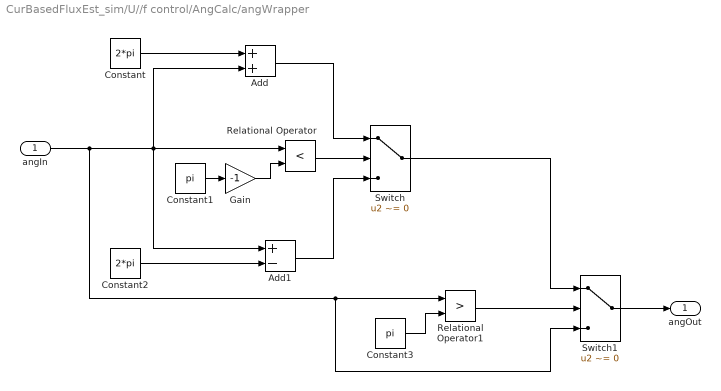
== system CurBasedFluxEst_sim/U//f control/AngCalc/angWrapper ==
  angIn : Inport
  Add : Sum
  Add1 : Sum  Inputs=+-
  Constant : Constant  Value=2*pi
  Constant1 : Constant  Value=pi
  Constant2 : Constant  Value=2*pi
  Constant3 : Constant  Value=pi
  Gain : Gain  Gain=-1
  Relational Operator : RelationalOperator  Operator=<  OutDataTypeStr=boolean  RndMeth=Simplest
  Relational Operator1 : RelationalOperator  Operator=>  OutDataTypeStr=boolean  RndMeth=Simplest
  Switch : Switch  Criteria=u2 ~= 0  Threshold=Ts_stair * NsCntr
  Switch1 : Switch  Criteria=u2 ~= 0  Threshold=Ts_stair * NsCntr
  angOut : Outport
  wires:
  angIn/1 -> Relational Operator1/1, Switch1/3, Relational Operator/1, Add/2, Add1/1
  Gain/1 -> Relational Operator/2
  Constant1/1 -> Gain/1
  Relational Operator/1 -> Switch/2
  Constant/1 -> Add/1
  Add/1 -> Switch/1
  Constant2/1 -> Add1/2
  Add1/1 -> Switch/3
  Switch/1 -> Switch1/1
  Relational Operator1/1 -> Switch1/2
  Constant3/1 -> Relational Operator1/2
  Switch1/1 -> angOut/1

== system CurBasedFluxEst_sim/U//f control/UAmpCalc/BelowFWPoint ==
  FreqRef : Inport
  UFWPoint : Inport  Port=2
  Add : Sum  Inputs=-+
  Add1 : Sum  Inputs=+-
  Add2 : Sum  Inputs=-+
  Add3 : Sum
  Divide : Product  Inputs=*/
  Product : Product
  UFCtrl_FWPointFreq : Constant  Value=UFCtrl_FWPointFreq
  UFCtrl_LinRegPointFreq : Constant  Value=UFCtrl_LinRegPointFreq
  UFCtrl_UBelowLinReg : Constant  Value=UFCtrl_UBelowLinReg
  Uamp : Outport
  wires:
  Add/1 -> Divide/1
  UFCtrl_LinRegPointFreq/1 -> Add1/2, Add2/1
  UFCtrl_UBelowLinReg/1 -> Add/1, Add3/1
  Product/1 -> Add3/2
  Divide/1 -> Product/1
  UFCtrl_FWPointFreq/1 -> Add1/1
  Add1/1 -> Divide/2
  Add2/1 -> Product/2
  Add3/1 -> Uamp/1
  UFWPoint/1 -> Add/2
  FreqRef/1 -> Add2/2

== matlab function CurBasedFluxEst_sim/IRR_LPF/MATLAB Function ==
  data: alpha output; Fc input; Fs input
% Calculating alpha coefficient for first-order IRR lowpass-filter with 
% the given cutoff frequency.

% Fc - cutoff frequency ( gain = 1/sqrt(2) ) [Hz]
% Ff - fundamental frequency ( gain ≈ 1 )    [Hz]
% Fs - sampling frequency ( gain ≈ 0 )       [Hz]

function alpha  = CalcAlphaLpIRR(Fc,Fs)
   
    theta = 2 * pi *( Fc / Fs );
    c = cos(theta);
    alpha1 = ( -2 * c + 2  + sqrt( (2 * c - 2)^2 - 8*c + 8 ) ) / -2;
    alpha2 = ( -2 * c + 2  - sqrt( (2 * c - 2)^2 - 8*c + 8 ) ) / -2;

    if( abs(alpha1) > 0 && abs(alpha1) < 1 && abs(alpha1) < abs(alpha2))
        alpha = abs(alpha1);
    else
        alpha = abs(alpha2);
    end
   
end
